simulink model "SpectreFiniV2"  (R2015a)
settings: Solver=ode45  StartTime=0.0  StopTime=10.0  RelTol=1e-6
values from neighbouring files (symbols this model uses):
  ex1 = expm(m.ee(2).a*h)    [SpectreFini_script.m]
  h = lsim(m.ee,u,t)    [Modeles.m]    (also in Parametres.m = 0.06)
  K = 1.1    [Modeles.m]    (also in SpectreFini_script.m = ones(1,2))
undefined symbols (not defined in the file or in its folder): m
libraries: dspmtrx3 x2
settings Model: Creator=David  LastModifiedBy=David
settings DataIOCC: LimitDataPoints=off

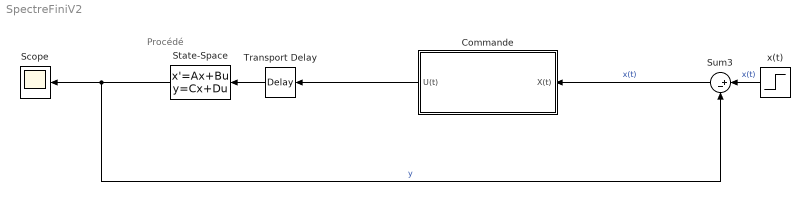
== system SpectreFiniV2 ==
  note: Procédé
  Commande : Subsystem
  Scope : Scope
  State-Space : StateSpace  A=m.ee(2).a  B=m.ee(2).b  C=m.ee(2).c  D=m.ee(2).d  X0=0
  Sum3 : Sum  Inputs=|+-
  Transport Delay : TransportDelay  DelayTime=h
  x(t) : Step  SampleTime=0
  wires:
  Transport Delay/1 -> State-Space/1
  State-Space/1 -> Sum3/2, Scope/1  "y"
  x(t)/1 -> Sum3/1  "x(t)"
  Sum3/1 -> Commande/1(X(t))  "x(t)"
  Commande/1(U(t)) -> Transport Delay/1

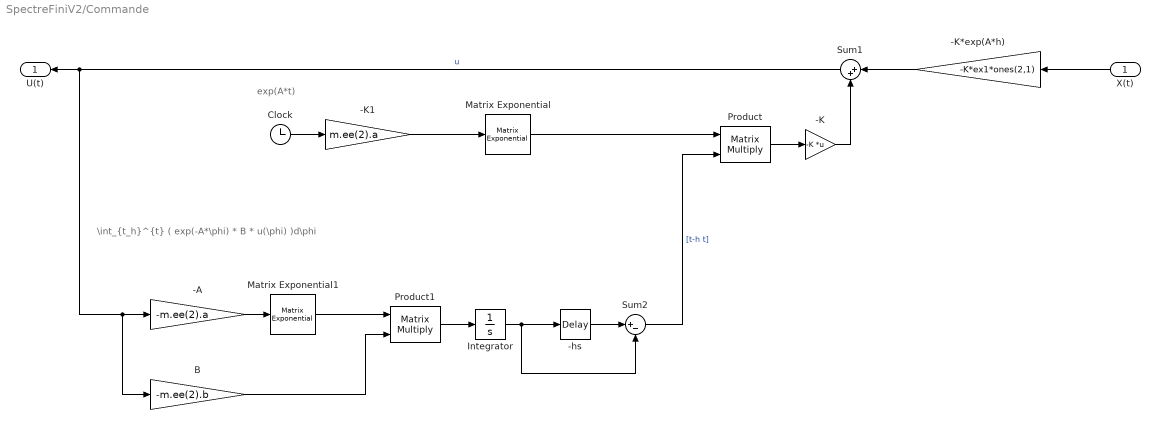
== system SpectreFiniV2/Commande ==
  note: \int_{t_h}^{t} ( exp(-A*\phi) * B * u(\phi) )d\phi
  note: exp(A*t)
  X(t) : Inport
  -A : Gain  Gain=-m.ee(2).a
  -K : Gain  Gain=-K  Multiplication=Matrix(K*u)
  -K*exp(A*h) : Gain  Gain=-K*ex1*ones(2,1)
  -K1 : Gain  Gain=m.ee(2).a
  -hs : TransportDelay  DelayTime=h
  B : Gain  Gain=-m.ee(2).b
  Clock : Clock
  Integrator : Integrator  AbsoluteTolerance=1e-6
  Matrix Exponential : dspmtrx3/Matrix Exponential
  Matrix Exponential1 : dspmtrx3/Matrix Exponential
  Product : Product  Multiplication=Matrix(*)
  Product1 : Product  Multiplication=Matrix(*)
  Sum1 : Sum  Inputs=|++
  Sum2 : Sum  Inputs=|+-
  U(t) : Outport
  wires:
  B/1 -> Product1/2
  Matrix Exponential1/1 -> Product1/1
  -K/1 -> Sum1/2
  X(t)/1 -> -K*exp(A*h)/1
  Sum1/1 -> U(t)/1, B/1, -A/1  "u"
  -K*exp(A*h)/1 -> Sum1/1
  -hs/1 -> Sum2/1
  Sum2/1 -> Product/2  "[t-h t]"
  Product1/1 -> Integrator/1
  Integrator/1 -> Sum2/2, -hs/1
  Matrix Exponential/1 -> Product/1
  Product/1 -> -K/1
  Clock/1 -> -K1/1
  -A/1 -> Matrix Exponential1/1
  -K1/1 -> Matrix Exponential/1
